simulink model "Linearly_Controlled_Dynamimcs_Model"  (R2017b)
settings: Solver=VariableStepAuto  StartTime=0.0  StopTime=10.0  RelTol=1e-3
settings Model: Creator=Jesus  LastModifiedBy=Jesus

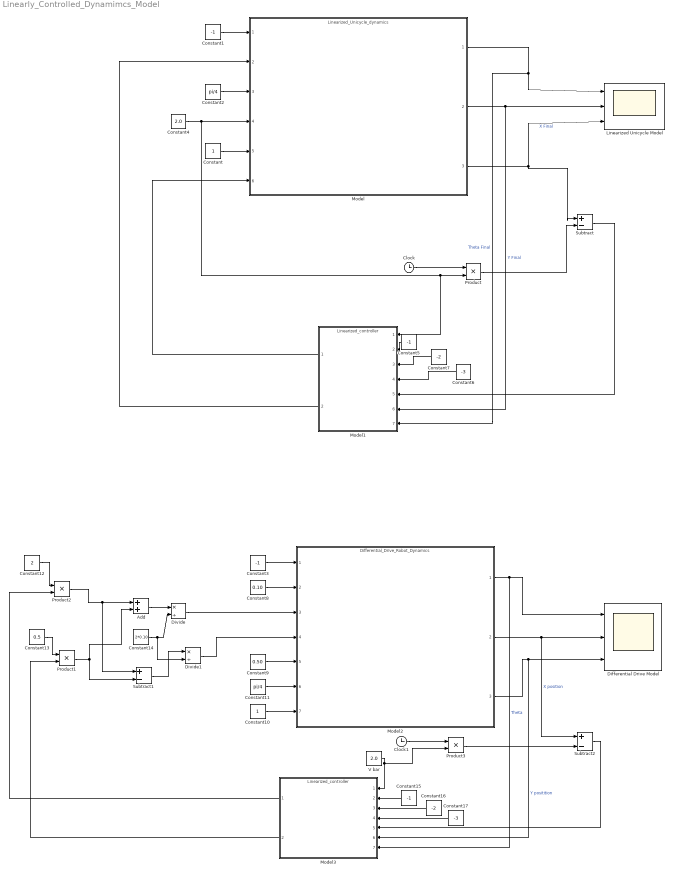
== system Linearly_Controlled_Dynamimcs_Model ==
  Add : Sum
  Clock : Clock
  Clock1 : Clock
  Constant : Constant
  Constant{1,3,5,15} (4 alike) : Constant  Value=-1
  Constant10 : Constant
  Constant11 : Constant  Value=pi/4
  Constant12 : Constant  Value=2
  Constant13 : Constant  Value=0.5
  Constant14 : Constant  Value=2*0.10
  Constant16 : Constant  Value=-2
  Constant17 : Constant  Value=-3
  Constant2 : Constant  Value=pi/4
  Constant4 : Constant  Value=2.0
  Constant6 : Constant  Value=-3
  Constant7 : Constant  Value=-2
  Constant8 : Constant  Value=0.10
  Constant9 : Constant  Value=0.50
  "Differential Drive Model " : Scope  NumInputPorts=3
  Divide : Product  Inputs=*/
  Divide1 : Product  Inputs=*/
  "Linearized Unicycle Model " : Scope  NumInputPorts=3
  Model : ModelReference  ModelNameDialog=Linearized_Unicycle_dynamics.slx  SimulationMode=Normal  ModelReferenceVersion=1.1
  Model1 : ModelReference  ModelNameDialog=Linearized_controller.slx  SimulationMode=Normal  ModelReferenceVersion=1.1
  Model2 : ModelReference  ModelNameDialog=Differential_Drive_Robot_Dynamics.slx  SimulationMode=Normal  ModelReferenceVersion=1.3
  Model3 : ModelReference  ModelNameDialog=Linearized_controller.slx  SimulationMode=Normal  ModelReferenceVersion=1.1
  Product{,1..3} (4 alike) : Product
  Subtract : Sum  Inputs=+-
  Subtract1 : Sum  Inputs=+-
  Subtract2 : Sum  Inputs=+-
  "V bar " : Constant  Value=2.0
  wires:
  Constant2/1 -> Model/3
  Constant1/1 -> Model/1
  Constant/1 -> Model/5
  Model/3 -> Subtract/1, "Linearized Unicycle Model "/3  "X Final"
  Model/2 -> Model1/6, "Linearized Unicycle Model "/2  "Y Final"
  Model/1 -> "Linearized Unicycle Model "/1, Model1/7  "Theta Final"
  Constant4/1 -> Model1/1, Product/2, Model/4
  Clock/1 -> Product/1
  Product/1 -> Subtract/2
  Subtract/1 -> Model1/5
  Constant5/1 -> Model1/2
  Constant7/1 -> Model1/3
  Constant6/1 -> Model1/4
  Model1/1 -> Model/6
  Model1/2 -> Model/2
  Constant11/1 -> Model2/6
  Constant3/1 -> Model2/1
  Model2/3 -> Model3/6, "Differential Drive Model "/3  "Y positition"
  Constant8/1 -> Model2/2
  Model3/2 -> Product1/2
  Constant13/1 -> Product1/1
  Product1/1 -> Add/2, Subtract1/2
  Constant9/1 -> Model2/5
  Add/1 -> Divide/1
  Model2/2 -> Subtract2/1, "Differential Drive Model "/2  "X position"
  Model2/1 -> Model3/7, "Differential Drive Model "/1  "Theta"
  Constant10/1 -> Model2/7
  Subtract1/1 -> Divide1/1
  Constant14/1 -> Divide1/2, Divide/2
  Divide1/1 -> Model2/4
  Divide/1 -> Model2/3
  Product2/1 -> Subtract1/1, Add/1
  Constant12/1 -> Product2/1
  Model3/1 -> Product2/2
  "V bar "/1 -> Product3/2, Model3/1
  Constant15/1 -> Model3/2
  Constant16/1 -> Model3/3
  Constant17/1 -> Model3/4
  Clock1/1 -> Product3/1
  Product3/1 -> Subtract2/2
  Subtract2/1 -> Model3/5
